simulink model "F_R_seat2019aversion"  (R2019a)
settings: Solver=FixedStepDiscrete  StartTime=0.0  StopTime=19  FixedStep=1  RelTol=1e-3
libraries: simulink x1
settings Model: Creator=A  LastModifiedBy=A

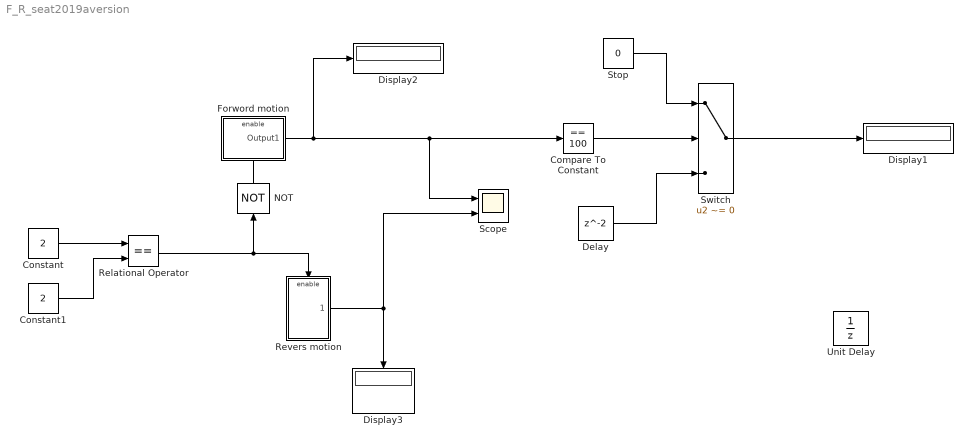
== system F_R_seat2019aversion ==
  Compare To Constant : simulink/Logic and Bit Operations/Compare To Constant  relop===  const=100  OutDataTypeStr=boolean
  Constant : Constant  Value=2
  Constant1 : Constant  Value=2
  Delay : Delay
  Display1 : Display
  Display2 : Display
  Display3 : Display
  Forword motion : Subsystem
  NOT : Logic  Operator=NOT  IconShape=distinctive  AllPortsSameDT=off  OutDataTypeStr=boolean
  Relational Operator : RelationalOperator  Operator===  OutDataTypeStr=boolean  RndMeth=Simplest
  Revers motion : Subsystem
  Scope : Scope  NumInputPorts=2
  Stop : Constant  Value=0
  Switch : Switch  Criteria=u2 ~= 0
  Unit Delay : UnitDelay  SampleTime=-1  HasFrameUpgradeWarning=on
  wires:
  Constant/1 -> Relational Operator/1
  Constant1/1 -> Relational Operator/2
  Relational Operator/1 -> Revers motion/Enable, NOT/1
  NOT/1 -> Forword motion/Enable
  Forword motion/1(Output1) -> Compare To Constant/1, Scope/1, Display2/1
  Revers motion/1(Output) -> Display3/1, Scope/2
  Compare To Constant/1 -> Switch/2
  Stop/1 -> Switch/1
  Switch/1 -> Display1/1
  Delay/1 -> Switch/3

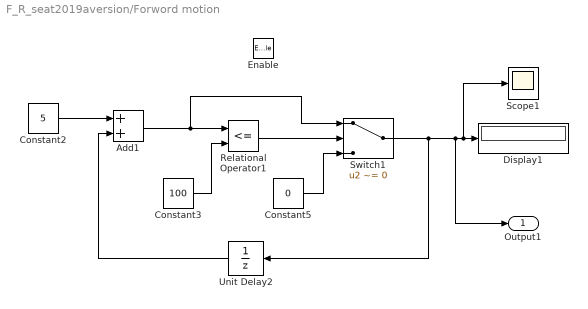
== system F_R_seat2019aversion/Forword motion ==
  Enable : EnablePort
  Add1 : Sum
  Constant2 : Constant  Value=5
  Constant3 : Constant  Value=100
  Constant5 : Constant  Value=0
  Display1 : Display
  Relational Operator1 : RelationalOperator  Operator=<=  OutDataTypeStr=boolean  RndMeth=Simplest
  Scope1 : Scope
  Switch1 : Switch  Criteria=u2 ~= 0
  Unit Delay2 : UnitDelay  InitialCondition=-1  SampleTime=-1  HasFrameUpgradeWarning=on
  Output1 : Outport
  wires:
  Unit Delay2/1 -> Add1/2
  Constant5/1 -> Switch1/3
  Relational Operator1/1 -> Switch1/2
  Constant2/1 -> Add1/1
  Add1/1 -> Switch1/1, Relational Operator1/1
  Switch1/1 -> Unit Delay2/1, Output1/1, Scope1/1, Display1/1
  Constant3/1 -> Relational Operator1/2

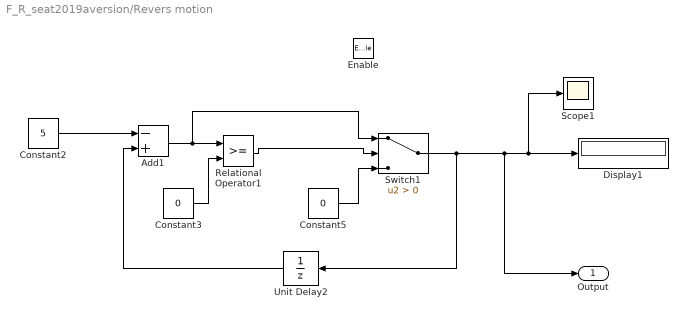
== system F_R_seat2019aversion/Revers motion ==
  Enable : EnablePort
  Add1 : Sum  Inputs=-+
  Constant2 : Constant  Value=5
  Constant3 : Constant  Value=0
  Constant5 : Constant  Value=0
  Display1 : Display
  Relational Operator1 : RelationalOperator  OutDataTypeStr=boolean  RndMeth=Simplest
  Scope1 : Scope
  Switch1 : Switch  Criteria=u2 > Threshold
  Unit Delay2 : UnitDelay  InitialCondition=100  SampleTime=-1  HasFrameUpgradeWarning=on
  Output : Outport
  wires:
  Relational Operator1/1 -> Switch1/2
  Constant2/1 -> Add1/1
  Constant5/1 -> Switch1/3
  Add1/1 -> Switch1/1, Relational Operator1/1
  Constant3/1 -> Relational Operator1/2
  Unit Delay2/1 -> Add1/2
  Switch1/1 -> Unit Delay2/1, Output/1, Display1/1, Scope1/1
